simulink model "gm_sampleModel1561_3_sub"  (R2023a)
settings: Solver=VariableStepAuto  StartTime=0.0  StopTime=10.0  RelTol=1e-3
libraries: simulink x2, hdlsllib x2
settings Model: Creator=user1  LastModifiedBy=user1
settings OptimizationCC: BlockReduction=off  ConditionallyExecuteInputs=off
settings DebuggingCC: InheritedTsInSrcMsg=none

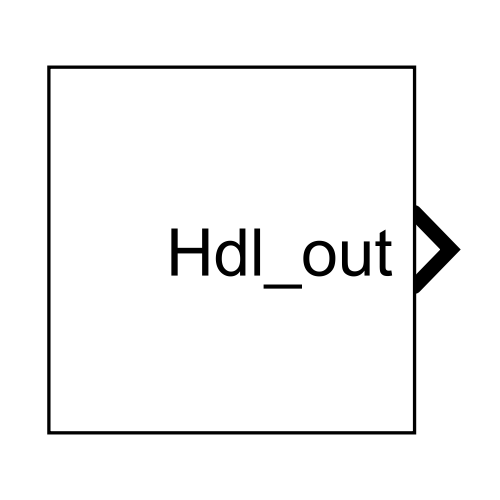
[thumbnail: Simulink's stored preview of the top-level diagram]
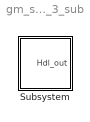
== system gm_sampleModel1561_3_sub ==
  Subsystem : Subsystem

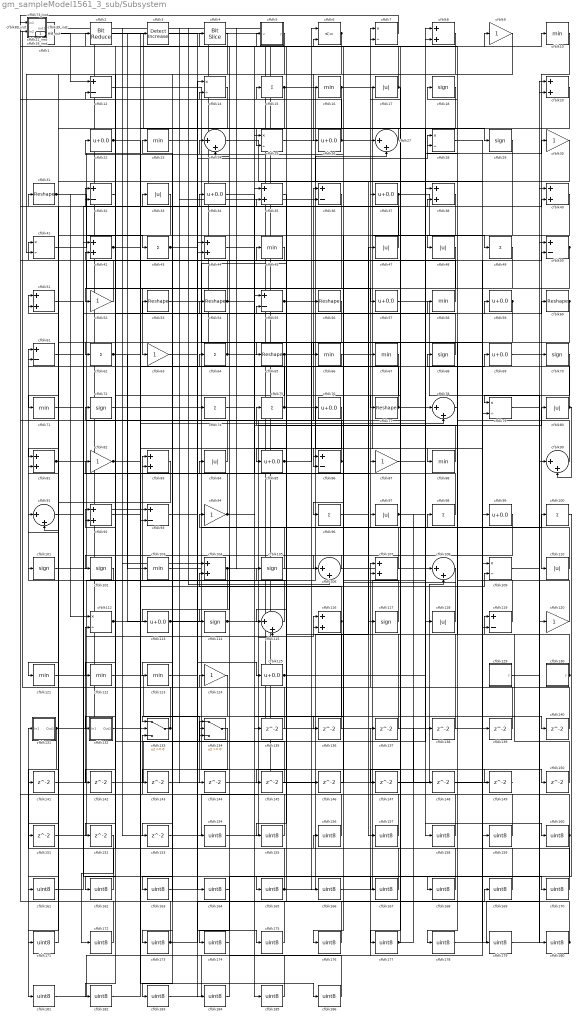
== system gm_sampleModel1561_3_sub/Subsystem ==
  cfblk1 : simulink/Logic and Bit Operations/Bit Set  iBit=0
      settings: LibrarySourceBlock=|
      | hdlsllib/Logic and Bit
      | Operations/Bit Set
  cfblk{10,16,23,45,58,66..67,71,88,103,121..123} (13 alike) : MinMax  OutDataTypeStr=uint8
  cfblk{15,43,49,62,64,74..75,96,98,100} (10 alike) : Sum  Inputs=+  OutDataTypeStr=uint8
  cfblk{18,29,68,70,72,101..102,105,114,117} (10 alike) : Signum
  cfblk{8,20,35,38,40,42,44,51,81,83,92,104,107,116} (14 alike) : Sum  OutDataTypeStr=uint8
  cfblk{24,27,78,90..91,106,108,115} (8 alike) : Sum  Inputs=|++  OutDataTypeStr=uint8
  cfblk{7,14,25,28,41,79,109,112} (8 alike) : Product  Inputs=*/  OutDataTypeStr=uint8  RndMeth=Zero  SaturateOnIntegerOverflow=on
  cfblk{17,33,47..48,80,84,97,110,118} (9 alike) : Abs  OutDataTypeStr=uint8  SaturateOnIntegerOverflow=off
  cfblk{22,26,34,37,57,59,69,76,85,99,113,125} (12 alike) : Bias  Bias=0.0  SaturateOnIntegerOverflow=off
  cfblk{12,32,36,50,55,61,86,93,119} (9 alike) : Sum  Inputs=+-  OutDataTypeStr=uint8
  cfblk11_inst : Subsystem
  cfblk{9,30,52,63,82,87,94,120,124} (9 alike) : Gain  OutDataTypeStr=uint8
  cfblk129 : Subsystem  mask(Counter Limited){uplimit=double(7), tsamp=double(-1)}
      mask prompts: uplimit "Simulink:masks:UpperLimit_MP"; tsamp "Simulink:masks:SampleTime_MP"
      mask help: Simulink:masks:CounterLimited_MD
      mask init:
      | nbits = double(8);
      | tsamp = double(-1);
      | uplimit = double(7);
  cfblk130 : Subsystem  mask(Counter Free-Running){NumBits=double(16), tsamp=double(-1)}
      mask prompts: NumBits "Simulink:masks:NumberOfBits_MP"; tsamp "Simulink:masks:SampleTime_MP"
      mask help: Simulink:masks:CounterFreeRunning_MD
  cfblk131 : Subsystem
  cfblk132 : Subsystem
  cfblk133 : Switch  OutDataTypeStr=uint8  SaturateOnIntegerOverflow=off  InputSameDT=off
  cfblk134 : Switch  OutDataTypeStr=uint8  SaturateOnIntegerOverflow=off  InputSameDT=off
  cfblk{135..153} (19 alike) : Delay  SampleTime=1
  cfblk13_inst : Subsystem
  cfblk{154..186} (33 alike) : DataTypeConversion  OutDataTypeStr=uint8  SaturateOnIntegerOverflow=off  RndMeth=Floor
  cfblk19_inst : Subsystem
  cfblk2 : hdlsllib/Logic and Bit Operations/Bit Reduce  mode=AND
  cfblk21_inst : Subsystem
  cfblk3 : simulink/Logic and Bit Operations/Detect Increase  vinit=0.0  OutDataTypeStr=uint8
      settings: LibrarySourceBlock=|
      | hdlsllib/Logic and Bit
      | Operations/Detect
      | Increase
  cfblk{31,53..54,56,60,65,77} (7 alike) : Reshape
  cfblk39_inst : Subsystem
  cfblk4 : hdlsllib/Logic and Bit Operations/Bit Slice  lidx=7  ridx=0
  cfblk5 : Subsystem  mask(Compare To Constant){relop=<=, const=double(3), OutDataTypeStr=uint8, ZeroCross=on}
      mask prompts: relop "Simulink:masks:Operator_MP"; const "Simulink:masks:ConstantValue_MP"; OutDataTypeStr "Simulink:masks:OutputDataType_MP"; ZeroCross "Simulink:masks:EnableZerocrossingDetection_MP"
      mask help: Simulink:masks:CompareToConstant_MD
      mask init:
      | OutDataTypeStr = 'uint8';
      | ZeroCross = 'on';
      | blkName = 'sampleModel1561_3_sub/Subsystem/cfblk5';
      | const = double(3);
      | const_str = '3.0';
      | const_val = double(3);
      | relop = '<=';
      | setValue = 'fixdt(0, 8)';
      | str = '<= 3';
      mask TypeOptions relop: == | ~= | < | <= | >= | >
      mask TypeOptions OutDataTypeStr: Simulink:masks:uint8 | Simulink:masks:boolean
      mask Callback ZeroCross: sl('zeroCrossEnable', gcbh);
      mask Display: disp(str)
  cfblk6 : RelationalOperator  Operator=<=  OutDataTypeStr=boolean  InputSameDT=off
  cfblk73_inst : Subsystem
  cfblk89_inst : Subsystem
  Hdl_out : Outport  OutDataTypeStr=uint8  SampleTime=1
  wires:
  cfblk1/1 -> cfblk12/1
  cfblk10/1 -> cfblk110/1
  cfblk100/1 -> cfblk165/1
  cfblk101/1 -> cfblk45/1
  cfblk102/1 -> cfblk61/1
  cfblk103/1 -> cfblk35/2
  cfblk104/1 -> cfblk113/1, cfblk98/1
  cfblk105/1 -> cfblk94/1
  cfblk106/1 -> cfblk102/1
  cfblk107/1 -> cfblk64/1
  cfblk108/1 -> cfblk107/1
  cfblk109/1 -> cfblk180/1
  cfblk11_inst/1(out1) -> cfblk133/2, cfblk106/2, cfblk139/1
  cfblk110/1 -> cfblk7/1
  cfblk112/1 -> cfblk78/2, cfblk69/1, cfblk55/2
  cfblk113/1 -> cfblk97/1, cfblk149/1
  cfblk114/1 -> cfblk80/1, Hdl_out/1
  cfblk115/1 -> cfblk83/1
  cfblk116/1 -> cfblk163/1, cfblk104/2
  cfblk117/1 -> cfblk22/1
  cfblk118/1 -> cfblk72/1
  cfblk119/1 -> cfblk5/1(u)
  cfblk12/1 -> cfblk79/2
  cfblk120/1 -> cfblk75/1
  cfblk121/1 -> cfblk27/2
  cfblk122/1 -> cfblk144/1
  cfblk123/1 -> cfblk44/1
  cfblk124/1 -> cfblk173/1
  cfblk125/1 -> cfblk8/2, cfblk15/1
  cfblk129/1(y) -> cfblk70/1
  cfblk13_inst/1(out1) -> cfblk108/1
  cfblk130/1(y) -> cfblk101/1, cfblk28/1
  cfblk131/1(Out1) -> cfblk40/2, cfblk181/1
  cfblk132/1(Out1) -> cfblk116/1
  cfblk133/1 -> cfblk91/2, cfblk91/1
  cfblk134/1 -> cfblk183/1
  cfblk135/1 -> cfblk13_inst/2(in2)
  cfblk136/1 -> cfblk73_inst/1(in1)
  cfblk137/1 -> cfblk83/2
  cfblk138/1 -> cfblk39_inst/2(in2)
  cfblk139/1 -> cfblk107/2
  cfblk14/1 -> cfblk162/1
  cfblk140/1 -> cfblk81/2
  cfblk141/1 -> cfblk112/2
  cfblk142/1 -> cfblk78/1
  cfblk143/1 -> cfblk164/1
  cfblk144/1 -> cfblk36/1
  cfblk145/1 -> cfblk12/2
  cfblk146/1 -> cfblk6/2
  cfblk147/1 -> cfblk108/2
  cfblk148/1 -> cfblk50/2
  cfblk149/1 -> cfblk1/1
  cfblk15/1 -> cfblk159/1, cfblk52/1
  cfblk150/1 -> cfblk119/1
  cfblk151/1 -> cfblk116/2
  cfblk152/1 -> cfblk172/1
  cfblk153/1 -> cfblk115/2
  cfblk154/1 -> cfblk6/1
  cfblk155/1 -> cfblk21_inst/1(in1)
  cfblk156/1 -> cfblk21_inst/2(in2)
  cfblk157/1 -> cfblk41/1
  cfblk158/1 -> cfblk24/1
  cfblk159/1 -> cfblk24/2
  cfblk16/1 -> cfblk133/1, cfblk88/1
  cfblk160/1 -> cfblk174/1, cfblk133/3
  cfblk161/1 -> cfblk87/1
  cfblk162/1 -> cfblk31/1
  cfblk163/1 -> cfblk14/1
  cfblk164/1 -> cfblk14/2
  cfblk165/1 -> cfblk47/1, cfblk131/1(In1)
  cfblk166/1 -> cfblk100/1
  cfblk167/1 -> cfblk156/1
  cfblk168/1 -> cfblk92/1
  cfblk169/1 -> cfblk92/2
  cfblk17/1 -> cfblk77/1, cfblk19_inst/1(in1)
  cfblk170/1 -> cfblk84/1
  cfblk171/1 -> cfblk51/1
  cfblk172/1 -> cfblk51/2
  cfblk173/1 -> cfblk73_inst/2(in2), cfblk169/1
  cfblk174/1 -> cfblk124/1
  cfblk175/1 -> cfblk89_inst/1(in1)
  cfblk176/1 -> cfblk23/1
  cfblk177/1 -> cfblk7/2, cfblk138/1
  cfblk178/1 -> cfblk20/1
  cfblk179/1 -> cfblk20/2
  cfblk18/1 -> cfblk121/1
  cfblk180/1 -> cfblk89_inst/2(in2), cfblk17/1, cfblk105/1
  cfblk181/1 -> cfblk109/1
  cfblk182/1 -> cfblk109/2
  cfblk183/1 -> cfblk137/1
  cfblk184/1 -> cfblk134/1
  cfblk185/1 -> cfblk134/2
  cfblk186/1 -> cfblk134/3
  cfblk19_inst/1(out1) -> cfblk104/1, cfblk146/1
  cfblk2/1 -> cfblk118/1
  cfblk20/1 -> cfblk177/1
  cfblk21_inst/1(out1) -> cfblk154/1
  cfblk22/1 -> cfblk29/1, cfblk186/1
  cfblk23/1 -> cfblk175/1
  cfblk24/1 -> cfblk157/1
  cfblk25/1 -> cfblk117/1
  cfblk26/1 -> cfblk99/1, cfblk19_inst/2(in2)
  cfblk27/1 -> cfblk25/2
  cfblk28/1 -> cfblk150/1
  cfblk29/1 -> cfblk48/1
  cfblk3/1 -> cfblk44/2
  cfblk30/1 -> cfblk71/1
  cfblk31/1 -> cfblk135/1, cfblk112/1, cfblk43/1, cfblk74/1
  cfblk32/1 -> cfblk2/1
  cfblk33/1 -> cfblk122/1
  cfblk34/1 -> cfblk57/1
  cfblk35/1 -> cfblk85/1
  cfblk36/1 -> cfblk63/1
  cfblk37/1 -> cfblk152/1, cfblk151/1, cfblk49/1
  cfblk38/1 -> cfblk123/1
  cfblk39_inst/1(out1) -> cfblk36/2
  cfblk4/1 -> cfblk143/1
  cfblk40/1 -> cfblk176/1
  cfblk41/1 -> cfblk3/1
  cfblk42/1 -> cfblk86/2, cfblk37/1
  cfblk43/1 -> cfblk125/1, cfblk153/1
  cfblk44/1 -> cfblk140/1
  cfblk45/1 -> cfblk42/2
  cfblk47/1 -> cfblk13_inst/1(in1)
  cfblk48/1 -> cfblk96/1
  cfblk49/1 -> cfblk155/1
  cfblk5/1(y) -> cfblk132/1(In1)
  cfblk50/1 -> cfblk119/2, cfblk62/1
  cfblk51/1 -> cfblk170/1
  cfblk52/1 -> cfblk42/1
  cfblk53/1 -> cfblk166/1
  cfblk54/1 -> cfblk11_inst/2(in2), cfblk66/1
  cfblk55/1 -> cfblk38/2, cfblk145/1
  cfblk56/1 -> cfblk161/1
  cfblk57/1 -> cfblk90/1
  cfblk58/1 -> cfblk4/1
  cfblk59/1 -> cfblk106/1, cfblk141/1
  cfblk6/1 -> cfblk81/1, cfblk41/2
  cfblk60/1 -> cfblk65/1, cfblk178/1
  cfblk61/1 -> cfblk38/1
  cfblk62/1 -> cfblk54/1, cfblk103/1
  cfblk63/1 -> cfblk50/1
  cfblk64/1 -> cfblk56/1, cfblk32/1
  cfblk65/1 -> cfblk182/1, cfblk142/1
  cfblk66/1 -> cfblk61/2
  cfblk67/1 -> cfblk115/1
  cfblk68/1 -> cfblk33/1
  cfblk69/1 -> cfblk40/1
  cfblk7/1 -> cfblk11_inst/1(in1)
  cfblk70/1 -> cfblk79/1
  cfblk71/1 -> cfblk34/1
  cfblk72/1 -> cfblk184/1
  cfblk73_inst/1(out1) -> cfblk67/1
  cfblk74/1 -> cfblk8/1
  cfblk75/1 -> cfblk53/1, cfblk179/1
  cfblk76/1 -> cfblk86/1
  cfblk77/1 -> cfblk55/1, cfblk30/1
  cfblk78/1 -> cfblk168/1
  cfblk79/1 -> cfblk120/1
  cfblk8/1 -> cfblk26/1
  cfblk80/1 -> cfblk90/2, cfblk18/1
  cfblk81/1 -> cfblk76/1, cfblk60/1
  cfblk82/1 -> cfblk93/2, cfblk9/1
  cfblk83/1 -> cfblk171/1
  cfblk84/1 -> cfblk39_inst/1(in1)
  cfblk85/1 -> cfblk28/2, cfblk10/1
  cfblk86/1 -> cfblk32/2, cfblk136/1
  cfblk87/1 -> cfblk160/1
  cfblk88/1 -> cfblk25/1
  cfblk89_inst/1(out1) -> cfblk93/1
  cfblk9/1 -> cfblk16/1
  cfblk90/1 -> cfblk68/1
  cfblk91/1 -> cfblk59/1
  cfblk92/1 -> cfblk167/1
  cfblk93/1 -> cfblk27/1
  cfblk94/1 -> cfblk185/1, cfblk82/1
  cfblk96/1 -> cfblk58/1
  cfblk97/1 -> cfblk158/1, cfblk148/1, cfblk147/1
  cfblk98/1 -> cfblk35/1
  cfblk99/1 -> cfblk114/1

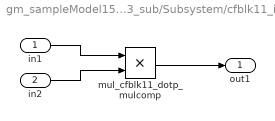
== system gm_sampleModel1561_3_sub/Subsystem/cfblk11_inst ==
  in1 : Inport  OutDataTypeStr=uint8  SampleTime=1
  in2 : Inport  Port=2  OutDataTypeStr=uint8  SampleTime=1
  mul_cfblk11_dotp_mulcomp : Product  Inputs=**  OutDataTypeStr=uint8  SampleTime=1
  out1 : Outport  OutDataTypeStr=uint8  SampleTime=1
  wires:
  in1/1 -> mul_cfblk11_dotp_mulcomp/1
  in2/1 -> mul_cfblk11_dotp_mulcomp/2
  mul_cfblk11_dotp_mulcomp/1 -> out1/1

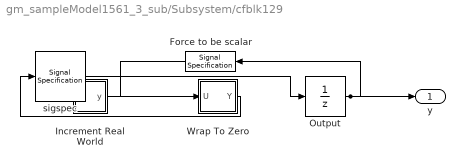
== system gm_sampleModel1561_3_sub/Subsystem/cfblk129 ==
  Force to be scalar : SignalSpecification  DisableCoverage=on  Dimensions=1
  Increment Real World : Subsystem  mask(Real World Value Increment){}
      mask help: Simulink:masks:RealWorldValueIncrement_MD
      mask Display: disp('V++')
  Output : UnitDelay  InitialCondition=0.0  SampleTime=tsamp  HasFrameUpgradeWarning=on
  Wrap To Zero : Subsystem  mask(Wrap To Zero){Threshold=double(7)}
      mask prompts: Threshold "Simulink:masks:Threshold_MP"
      mask help: Simulink:masks:WrapToZero_MD
  sigspec : SignalSpecification  OutDataTypeStr=uint8  Dimensions=1
  y : Outport  SampleTime=1
  wires:
  Force to be scalar/1 -> Increment Real World/1(u)
  Increment Real World/1(y) -> Wrap To Zero/1(U)
  Output/1 -> Force to be scalar/1, y/1
  Wrap To Zero/1(Y) -> sigspec/1
  sigspec/1 -> Output/1

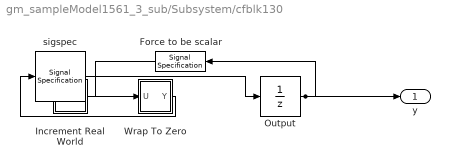
== system gm_sampleModel1561_3_sub/Subsystem/cfblk130 ==
  Force to be scalar : SignalSpecification  DisableCoverage=on  Dimensions=1
  Increment Real World : Subsystem  mask(Real World Value Increment){}
      mask help: Simulink:masks:RealWorldValueIncrement_MD
      mask Display: disp('V++')
  Output : UnitDelay  InitialCondition=0.0  SampleTime=tsamp  HasFrameUpgradeWarning=on
  Wrap To Zero : Subsystem  mask(Wrap To Zero){Threshold=double(65535)}
      mask prompts: Threshold "Simulink:masks:Threshold_MP"
      mask help: Simulink:masks:WrapToZero_MD
  sigspec : SignalSpecification  OutDataTypeStr=uint16  Dimensions=1
  y : Outport  SampleTime=1
  wires:
  Force to be scalar/1 -> Increment Real World/1(u)
  Increment Real World/1(y) -> Wrap To Zero/1(U)
  Output/1 -> Force to be scalar/1, y/1
  Wrap To Zero/1(Y) -> sigspec/1
  sigspec/1 -> Output/1

== system gm_sampleModel1561_3_sub/Subsystem/cfblk131 ==
  In1 : Inport  OutDataTypeStr=uint8  PortDimensions=1  SampleTime=1
  Out1 : Outport  SampleTime=1
  wires:
  In1/1 -> Out1/1

== system gm_sampleModel1561_3_sub/Subsystem/cfblk132 ==
  In1 : Inport  OutDataTypeStr=uint8  PortDimensions=1  SampleTime=1
  Out1 : Outport  SampleTime=1
  wires:
  In1/1 -> Out1/1

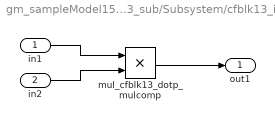
== system gm_sampleModel1561_3_sub/Subsystem/cfblk13_inst ==
  in1 : Inport  OutDataTypeStr=uint8  SampleTime=1
  in2 : Inport  Port=2  OutDataTypeStr=uint8  SampleTime=1
  mul_cfblk13_dotp_mulcomp : Product  Inputs=**  OutDataTypeStr=uint8  SampleTime=1
  out1 : Outport  OutDataTypeStr=uint8  SampleTime=1
  wires:
  in1/1 -> mul_cfblk13_dotp_mulcomp/1
  in2/1 -> mul_cfblk13_dotp_mulcomp/2
  mul_cfblk13_dotp_mulcomp/1 -> out1/1

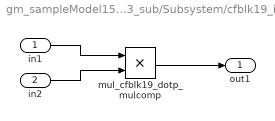
== system gm_sampleModel1561_3_sub/Subsystem/cfblk19_inst ==
  in1 : Inport  OutDataTypeStr=uint8  SampleTime=1
  in2 : Inport  Port=2  OutDataTypeStr=uint8  SampleTime=1
  mul_cfblk19_dotp_mulcomp : Product  Inputs=**  OutDataTypeStr=uint8  SampleTime=1
  out1 : Outport  OutDataTypeStr=uint8  SampleTime=1
  wires:
  in1/1 -> mul_cfblk19_dotp_mulcomp/1
  in2/1 -> mul_cfblk19_dotp_mulcomp/2
  mul_cfblk19_dotp_mulcomp/1 -> out1/1

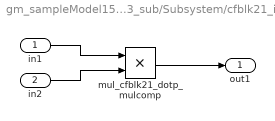
== system gm_sampleModel1561_3_sub/Subsystem/cfblk21_inst ==
  in1 : Inport  OutDataTypeStr=uint8  SampleTime=1
  in2 : Inport  Port=2  OutDataTypeStr=uint8  SampleTime=1
  mul_cfblk21_dotp_mulcomp : Product  Inputs=**  OutDataTypeStr=uint8  SampleTime=1
  out1 : Outport  OutDataTypeStr=uint8  SampleTime=1
  wires:
  in1/1 -> mul_cfblk21_dotp_mulcomp/1
  in2/1 -> mul_cfblk21_dotp_mulcomp/2
  mul_cfblk21_dotp_mulcomp/1 -> out1/1

== system gm_sampleModel1561_3_sub/Subsystem/cfblk39_inst ==
  in1 : Inport  OutDataTypeStr=uint8  SampleTime=1
  in2 : Inport  Port=2  OutDataTypeStr=uint8  SampleTime=1
  mul_cfblk39_dotp_mulcomp : Product  Inputs=**  OutDataTypeStr=uint8  SampleTime=1
  out1 : Outport  OutDataTypeStr=uint8  SampleTime=1
  wires:
  in1/1 -> mul_cfblk39_dotp_mulcomp/1
  in2/1 -> mul_cfblk39_dotp_mulcomp/2
  mul_cfblk39_dotp_mulcomp/1 -> out1/1

== system gm_sampleModel1561_3_sub/Subsystem/cfblk5 ==
  u : Inport  OutDataTypeStr=uint8  SampleTime=1
  Compare : RelationalOperator  Operator=<=  OutDataTypeStr=fixdt(0, 8)
  Constant : Constant  DisableCoverage=on  Value=const  OutDataTypeStr=Inherit: Inherit via back propagation  SampleTime=-1
  y : Outport  SampleTime=1
  wires:
  u/1 -> Compare/1
  Compare/1 -> y/1
  Constant/1 -> Compare/2

== system gm_sampleModel1561_3_sub/Subsystem/cfblk73_inst ==
  in1 : Inport  OutDataTypeStr=uint8  SampleTime=1
  in2 : Inport  Port=2  OutDataTypeStr=uint8  SampleTime=1
  mul_cfblk73_dotp_mulcomp : Product  Inputs=**  OutDataTypeStr=uint8  SampleTime=1
  out1 : Outport  OutDataTypeStr=uint8  SampleTime=1
  wires:
  in1/1 -> mul_cfblk73_dotp_mulcomp/1
  in2/1 -> mul_cfblk73_dotp_mulcomp/2
  mul_cfblk73_dotp_mulcomp/1 -> out1/1

== system gm_sampleModel1561_3_sub/Subsystem/cfblk89_inst ==
  in1 : Inport  OutDataTypeStr=uint8  SampleTime=1
  in2 : Inport  Port=2  OutDataTypeStr=uint8  SampleTime=1
  mul_cfblk89_dotp_mulcomp : Product  Inputs=**  OutDataTypeStr=uint8  SampleTime=1
  out1 : Outport  OutDataTypeStr=uint8  SampleTime=1
  wires:
  in1/1 -> mul_cfblk89_dotp_mulcomp/1
  in2/1 -> mul_cfblk89_dotp_mulcomp/2
  mul_cfblk89_dotp_mulcomp/1 -> out1/1

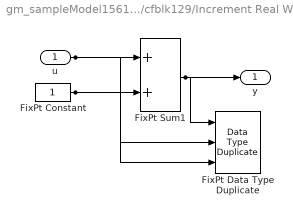
== system gm_sampleModel1561_3_sub/Subsystem/cfblk129/Increment Real World ==
  u : Inport  OutDataTypeStr=uint8  SampleTime=1
  FixPt Constant : Constant  DisableCoverage=on  OutDataTypeStr=Inherit: Inherit via back propagation  SampleTime=-1
  FixPt Data Type Duplicate : DataTypeDuplicate  DisableCoverage=on  NumInputPorts=3
  FixPt Sum1 : Sum  InputSameDT=on  OutDataTypeStr=Inherit: Inherit via back propagation  LockScale=on
  y : Outport  SampleTime=1
  wires:
  u/1 -> FixPt Sum1/1, FixPt Data Type Duplicate/2
  FixPt Constant/1 -> FixPt Sum1/2, FixPt Data Type Duplicate/3
  FixPt Sum1/1 -> FixPt Data Type Duplicate/1, y/1

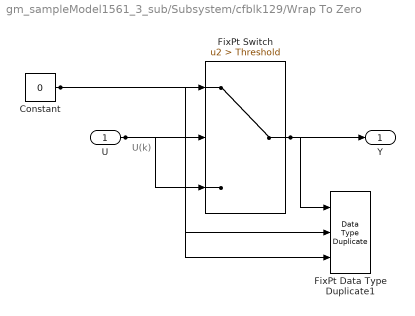
== system gm_sampleModel1561_3_sub/Subsystem/cfblk129/Wrap To Zero ==
  note: U(k)
  U : Inport  OutDataTypeStr=uint8  SampleTime=1
  Constant : Constant  DisableCoverage=on  Value=0  OutDataTypeStr=Inherit: Inherit via back propagation  SampleTime=-1
  FixPt Data Type Duplicate1 : DataTypeDuplicate  DisableCoverage=on  NumInputPorts=3
  FixPt Switch : Switch  Criteria=u2 > Threshold  Threshold=Threshold  OutDataTypeStr=Inherit: Inherit via back propagation  ZeroCross=off  SaturateOnIntegerOverflow=off  InputSameDT=off
  Y : Outport  SampleTime=1
  wires:
  U/1 -> FixPt Switch/3, FixPt Switch/2, FixPt Data Type Duplicate1/2
  Constant/1 -> FixPt Switch/1, FixPt Data Type Duplicate1/3
  FixPt Switch/1 -> FixPt Data Type Duplicate1/1, Y/1

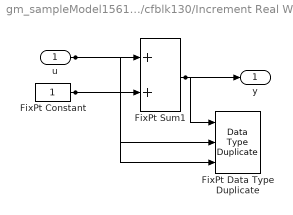
== system gm_sampleModel1561_3_sub/Subsystem/cfblk130/Increment Real World ==
  u : Inport  OutDataTypeStr=uint16  SampleTime=1
  FixPt Constant : Constant  DisableCoverage=on  OutDataTypeStr=Inherit: Inherit via back propagation  SampleTime=-1
  FixPt Data Type Duplicate : DataTypeDuplicate  DisableCoverage=on  NumInputPorts=3
  FixPt Sum1 : Sum  InputSameDT=on  OutDataTypeStr=Inherit: Inherit via back propagation  LockScale=on
  y : Outport  SampleTime=1
  wires:
  u/1 -> FixPt Sum1/1, FixPt Data Type Duplicate/2
  FixPt Constant/1 -> FixPt Sum1/2, FixPt Data Type Duplicate/3
  FixPt Sum1/1 -> FixPt Data Type Duplicate/1, y/1

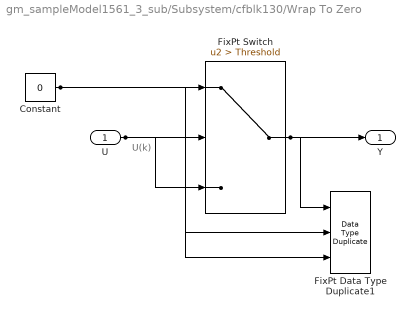
== system gm_sampleModel1561_3_sub/Subsystem/cfblk130/Wrap To Zero ==
  note: U(k)
  U : Inport  OutDataTypeStr=uint16  SampleTime=1
  Constant : Constant  DisableCoverage=on  Value=0  OutDataTypeStr=Inherit: Inherit via back propagation  SampleTime=-1
  FixPt Data Type Duplicate1 : DataTypeDuplicate  DisableCoverage=on  NumInputPorts=3
  FixPt Switch : Switch  Criteria=u2 > Threshold  Threshold=Threshold  OutDataTypeStr=Inherit: Inherit via back propagation  ZeroCross=off  SaturateOnIntegerOverflow=off  InputSameDT=off
  Y : Outport  SampleTime=1
  wires:
  U/1 -> FixPt Switch/3, FixPt Switch/2, FixPt Data Type Duplicate1/2
  Constant/1 -> FixPt Switch/1, FixPt Data Type Duplicate1/3
  FixPt Switch/1 -> FixPt Data Type Duplicate1/1, Y/1
